simulink model "exam2021_anti_simulink"  (R2022b)
settings: Solver=VariableStepAuto  StartTime=0.0  StopTime=50  RelTol=1e-3
settings Model: Creator=rohan  LastModifiedBy=Akash
settings DebuggingCC: UnconnectedInputMsg=warning  UnconnectedOutputMsg=warning  UnconnectedLineMsg=warning
settings ModelReferenceCC: EnableRefExpFcnMdlSchedulingChecks=on
settings RTWCC: DLArmComputeVersion=19.05

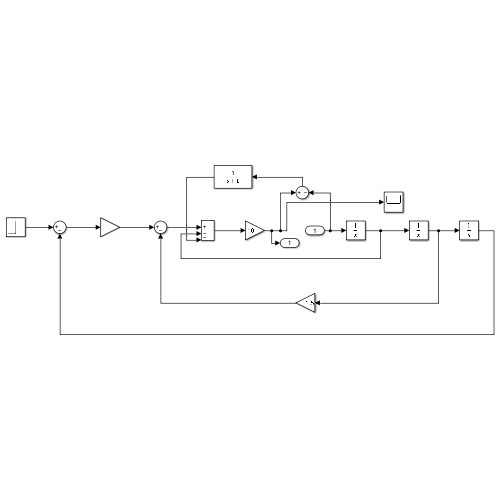
[thumbnail: Simulink's stored preview of the top-level diagram]
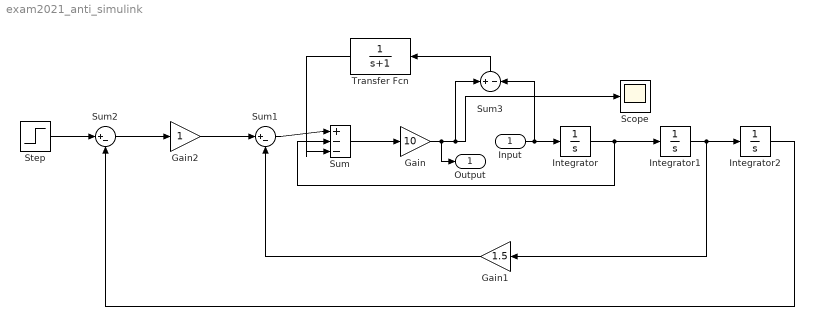
== system exam2021_anti_simulink ==
  Input : Inport
  Gain : Gain  Gain=10
  Gain1 : Gain  Gain=1.5
  Gain2 : Gain
  Integrator : Integrator
  Integrator1 : Integrator
  Integrator2 : Integrator
  Scope : Scope
  Step : Step  After=5.1  SampleTime=0
  Sum : Sum  Inputs=|+--
  Sum1 : Sum  Inputs=|+-
  Sum2 : Sum  Inputs=|+-
  Sum3 : Sum  Inputs=+-
  Transfer Fcn : TransferFcn  Denominator=[1 1]
  Output : Outport
  wires:
  Gain/1 -> Output/1, Sum3/1, Scope/1
  Sum/1 -> Gain/1
  Integrator/1 -> Integrator1/1, Sum/2
  Integrator1/1 -> Gain1/1, Integrator2/1
  Sum1/1 -> Sum/1
  Gain1/1 -> Sum1/2
  Gain2/1 -> Sum1/1
  Sum2/1 -> Gain2/1
  Integrator2/1 -> Sum2/2
  Step/1 -> Sum2/1
  Input/1 -> Sum3/2, Integrator/1
  Transfer Fcn/1 -> Sum/3
  Sum3/1 -> Transfer Fcn/1
